simulink model "MANCHESTER_Y"  (R2024b)
settings: Solver=VariableStepAuto  StartTime=0.0  StopTime=10.0  RelTol=1e-3
libraries: commrandsrc3 x1

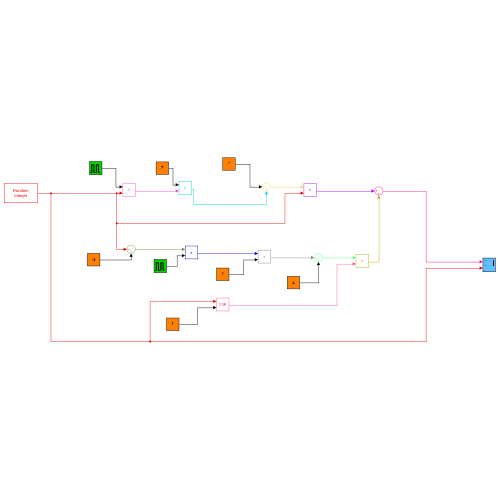
[thumbnail: Simulink's stored preview of the top-level diagram]
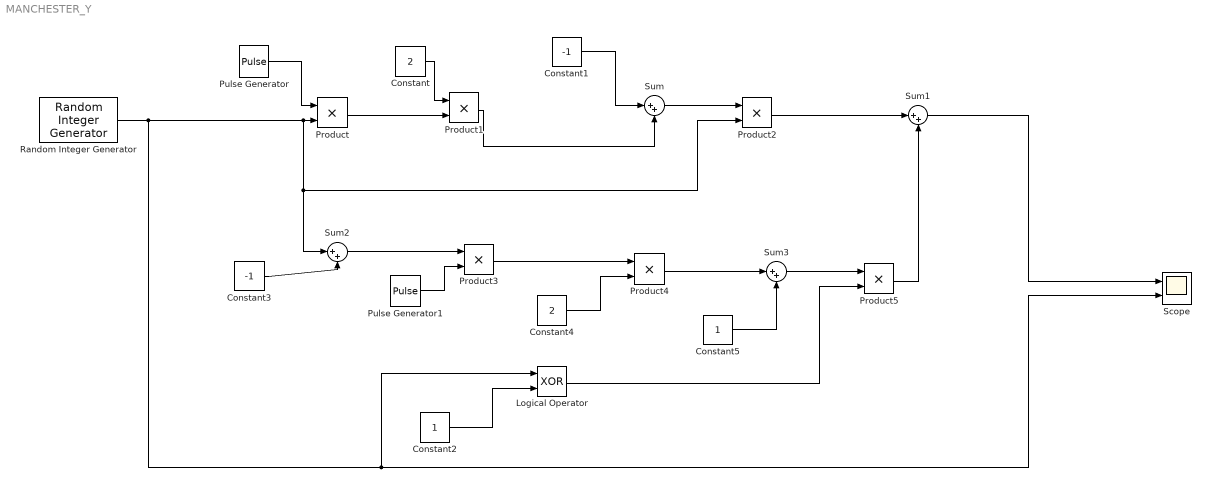
== system MANCHESTER_Y ==
  Constant : Constant  Value=2
  Constant1 : Constant  Value=-1
  Constant2 : Constant
  Constant3 : Constant  Value=-1
  Constant4 : Constant  Value=2
  Constant5 : Constant
  Logical Operator : Logic  Operator=XOR  AllPortsSameDT=off  OutDataTypeStr=boolean
  Product{,1..5} (6 alike) : Product
  Pulse Generator : DiscretePulseGenerator  PulseType=Time based  Period=0.1  PulseWidth=50
  Pulse Generator1 : DiscretePulseGenerator  PulseType=Time based  Period=0.1  PulseWidth=50
  Random Integer Generator : commrandsrc3/Random Integer Generator  SetSize=2  SeedSource=Auto  Seed=0  SampleTime=0.1  SamplesPerFrame=1  OutputDataType=double  SimulateUsing=Interpreted execution
  Scope : Scope  NumInputPorts=2
  Sum{,1..3} (4 alike) : Sum  Inputs=|++
  wires:
  Random Integer Generator/1 -> Product2/2, Sum2/1, Product/2, Logical Operator/1, Scope/2
  Pulse Generator/1 -> Product/1
  Product/1 -> Product1/2
  Constant/1 -> Product1/1
  Product1/1 -> Sum/2
  Constant1/1 -> Sum/1
  Sum/1 -> Product2/1
  Product2/1 -> Sum1/1
  Constant2/1 -> Logical Operator/2
  Constant3/1 -> Sum2/2
  Sum2/1 -> Product3/1
  Pulse Generator1/1 -> Product3/2
  Product3/1 -> Product4/1
  Constant4/1 -> Product4/2
  Constant5/1 -> Sum3/2
  Product4/1 -> Sum3/1
  Sum3/1 -> Product5/1
  Logical Operator/1 -> Product5/2
  Product5/1 -> Sum1/2
  Sum1/1 -> Scope/1
